simulink model "TVC_Control"  (R2025b)
settings: Solver=VariableStepAuto  StartTime=0.0  StopTime=12  RelTol=1e-3
libraries: simulink x1, simulink_extras x1
settings Model: Creator=HKARA  LastModifiedBy=HKARA

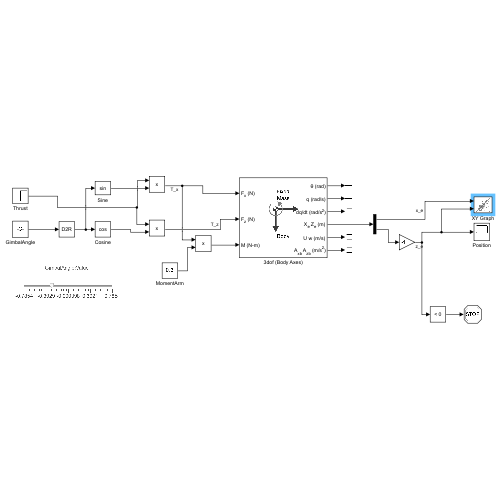
[thumbnail: Simulink's stored preview of the top-level diagram]
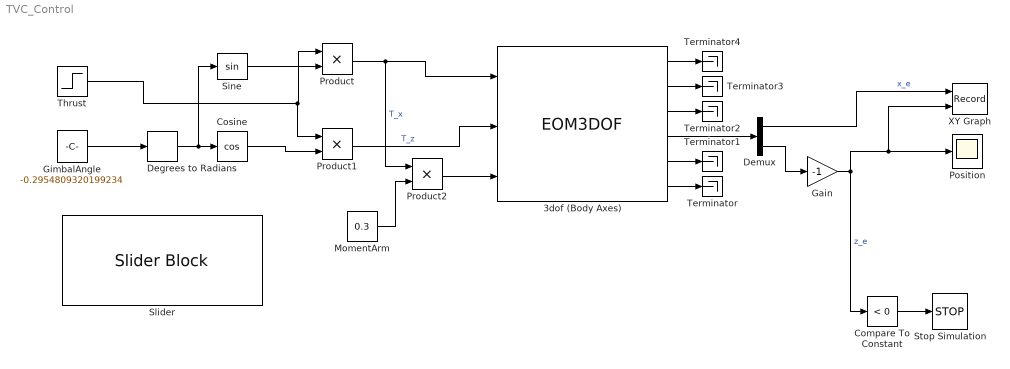
== system TVC_Control ==
  3dof (Body Axes) : EOM3DOF  v_ini=0  mass=0.55  Iyy=0.0448
  Compare To Constant : simulink/Logic and Bit Operations/Compare To Constant  relop=<  const=0  OutDataTypeStr=boolean
  Cosine : Trigonometry  Operator=cos
  Degrees to Radians : simulink_extras/Transformations/Degrees to Radians
  Demux : Demux  Outputs=2
  Gain : Gain  Gain=-1
  GimbalAngle : Constant  Value=-0.2954809320199234
  MomentArm : Constant  Value=0.3
  Position : Scope
      settings: ActiveDisplayYMinimum=-12.128174366282437  ActiveDisplayYMaximum=109.15349177934172
  Product : Product
  Product1 : Product
  Product2 : Product
  Sine : Trigonometry
  Slider : SliderBlock  ScaleMin=-0.785398  ScaleMax=0.785398
  Stop Simulation : Stop
  Terminator{,1..4} (5 alike) : Terminator
  Thrust : Step  Before=-15  After=0  SampleTime=2
  XY Graph : Record  NumPorts=2.0  FileSettingsInternal="{\"entries\":[{\"content\":{\"excelSettings\":{\"content\":{},\"type\":\"Streamout.ExcelSettings\"},\"parquetSettings\":{\"content\":{},\"type\":\"Streamout.ParquetSettings\"}},\"type\":\"Streamout.FileSettingStorage\",\"uuid\":\"\"}],\"packageUris\":[\"http:\\/\\/schema.mathworks.com\\/mf0\\/streamout_blocks\\/R2020a\"],\"version\":\"1.0\"}"  FrameSettings=[0, 0]  Layout=[1 1]  SignalsInternal="{\"entries\":[{\"content\":{\"signals\":[{\"content\":{\"blockPath\":[],\"dimensions\":[1],\"domain\":\"\",\"lineColor\":\"#a2142f\",\"plots\":[ 1 ],\"port\":1,\"sid\":[\"\"],\"signalID\":1,\"signalName\":\"x_e\"},\"type\":\"RecordBlkView.Signal\",\"uuid\":\"\"},{\"content\":{\"blockPath\":[],\"dimensions\":[1],\"domain\":\"\",\"lineColor\":\"#139fff\",\"plots\":[ 1 ],\"port\":2,\"sid\":[\"\"],\"signalID\":2,\"signalName\":\"z_e\"},\"type\":\"RecordBlkView.Signal\",\"uuid\":\"\"},{\"content\":{\"blockPath\":[],\"dimensions\":[1],\"domain\":\"\",\"lineColor\":\"#64d413\",\"lineWidth\":2,\"sid\":[\"\"],\"signalID\":3,\"signalName\":\"GimbalAngle:Value\"},\"type\":\"RecordBlkView.Signal\",\"uuid\":\"\"}]},\"type\":\"RecordBlkView.InputSignals\",\"uuid\":\"\"}],\"packageUris\":[\"http:\\/\\/schema.mathworks.com\\/mf0\\/streamout_blocks\\/R2020a\"],\"version\":\"1.0\"}"  VisualizationBindings="{\"xyplotplugin\":{\"info\":[{\"series\":[{\"bindingParametersList\":[{\"parameter\":\"X-Axis\",\"signalID\":1,\"signalName\":\"x_e\"},{\"parameter\":\"Y-Axis\",\"signalID\":2,\"signalName\":\"z_e\"},{\"parameter\":\"X-Axis\",\"signalID\":1,\"signalName\":\"x_e\"},{\"parameter\":\"Y-Axis\",\"signalID\":2,\"signalName\":\"z_e\"},{\"parameter\":\"X-Axis\",\"signalID\":1,\"signalName\":\"x_e\"},{\"parameter\":\"Y-Axis\",\"signalID\":2,\"signalName\":\"z_e\"},{\"parameter\":\"X-Axis\",\"signalID\":1,\"signalName\":\"x_e\"},{\"parameter\":\"Y-Axis\",\"signalID\":2,\"signalName\":\"z_e\"}],\"seriesID\":0}],\"subplotID\":1}]}}"  CompatibilityTag=XY
  wires:
  GimbalAngle/1 -> Degrees to Radians/1
  Degrees to Radians/1 -> Sine/1, Cosine/1
  Thrust/1 -> Product1/1, Product/1
  Cosine/1 -> Product1/2
  Sine/1 -> Product/2
  Product1/1 -> 3dof (Body Axes)/2  "T_z"
  MomentArm/1 -> Product2/2
  Product2/1 -> 3dof (Body Axes)/3
  Product/1 -> Product2/1, 3dof (Body Axes)/1  "T_x"
  3dof (Body Axes)/4 -> Demux/1
  Demux/1 -> XY Graph/1  "x_e"
  Demux/2 -> Gain/1
  Gain/1 -> Compare To Constant/1, XY Graph/2, Position/1  "z_e"
  Compare To Constant/1 -> Stop Simulation/1
  3dof (Body Axes)/6 -> Terminator/1
  3dof (Body Axes)/5 -> Terminator1/1
  3dof (Body Axes)/3 -> Terminator2/1
  3dof (Body Axes)/2 -> Terminator3/1
  3dof (Body Axes)/1 -> Terminator4/1
